simulink model "chap9_3sim"  (Simulink 3.00)
settings: Solver=ode45  StartTime=0.0  StopTime=30  RelTol=1e-3
settings Model: LastModifiedBy=liu

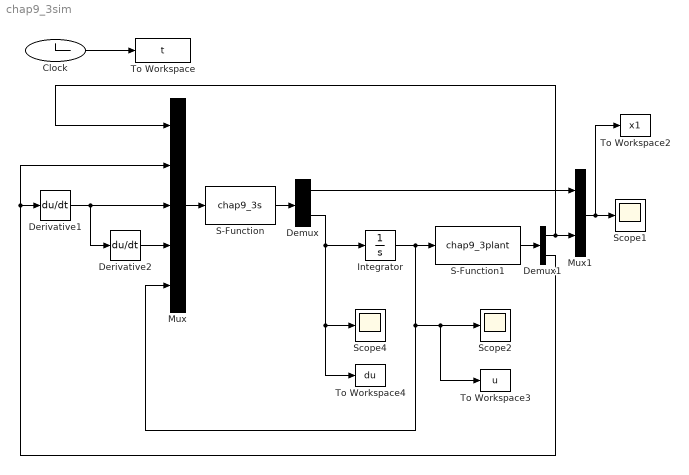
== system chap9_3sim ==
  Clock : Clock
  Demux : Demux  Outputs=2
  Demux1 : Demux  Outputs=2
  Derivative1 : Derivative
  Derivative2 : Derivative
  Integrator : Integrator  ExternalReset=none  InitialConditionSource=internal  InitialCondition=0  LimitOutput=off  UpperSaturationLimit=inf  LowerSaturationLimit=-inf  ShowSaturationPort=off  ShowStatePort=off  AbsoluteTolerance=auto
  Mux : Mux  Inputs=5
  Mux1 : Mux  Inputs=2
  S-Function : S-Function  FunctionName=chap9_3s  PortCounts=[]  SFunctionModules=''
  S-Function1 : S-Function  FunctionName=chap9_3plant  PortCounts=[]  SFunctionModules=''
  Scope1 : Scope
      settings: TimeRange=auto  YMin=-0.5  YMax=0.55  SaveToWorkspace=off  SaveName=ScopeData
  Scope2 : Scope
      settings: TimeRange=auto  YMin=-0.1665  YMax=-0.158  SaveToWorkspace=off  SaveName=ScopeData
  Scope4 : Scope
      settings: TimeRange=auto  YMin=-0.095  YMax=-0.015  SaveToWorkspace=off  SaveName=ScopeData
  To Workspace : ToWorkspace  VariableName=t  SampleTime=-1  SaveFormat=Matrix
  To Workspace2 : ToWorkspace  VariableName=x1  SampleTime=-1  SaveFormat=Matrix
  To Workspace3 : ToWorkspace  VariableName=u  SampleTime=-1  SaveFormat=Matrix
  To Workspace4 : ToWorkspace  VariableName=du  SampleTime=-1  SaveFormat=Matrix
  wires:
  Mux/1 -> S-Function/1
  Derivative2/1 -> Mux/4
  Integrator/1 -> S-Function1/1, Mux/5, Scope2/1, To Workspace3/1
  S-Function1/1 -> Demux1/1
  S-Function/1 -> Demux/1
  Demux/2 -> Integrator/1, Scope4/1, To Workspace4/1
  Derivative1/1 -> Mux/3, Derivative2/1
  Demux1/1 -> Mux1/2, Mux/1
  Demux1/2 -> Derivative1/1, Mux/2
  Demux/1 -> Mux1/1
  Mux1/1 -> To Workspace2/1, Scope1/1
  Clock/1 -> To Workspace/1
